simulink model "FeedForward_control"  (R2021a)
settings: Solver=VariableStepAuto  StartTime=0.0  StopTime=12.0  FixedStep=0.0001  MaxStep=0.1111111111111111  RelTol=1e-3
undefined symbols (not defined in the file): sigbuilder_block
settings Model: Creator=Mehra  LastModifiedBy=Mehra

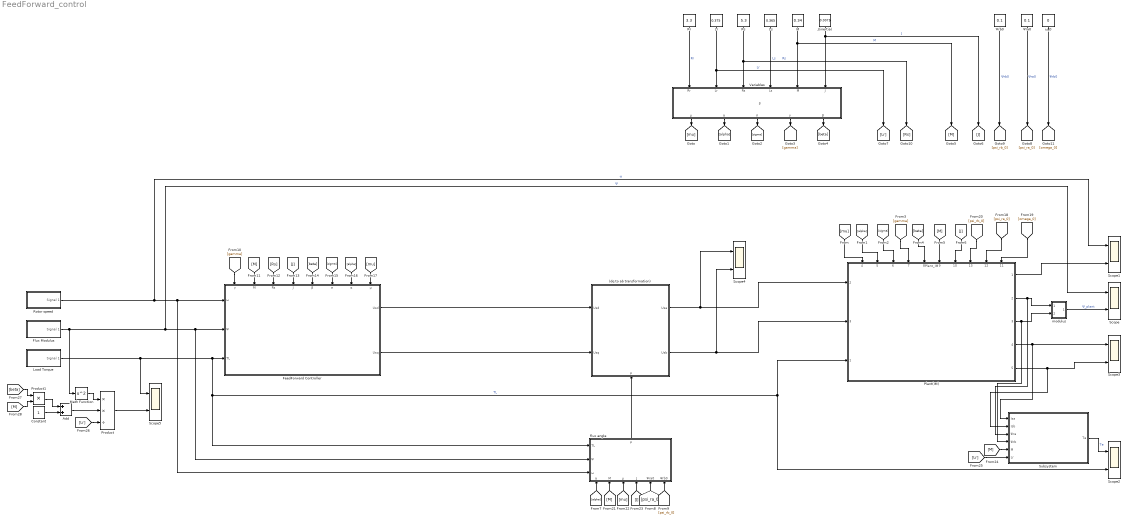
== system FeedForward_control ==
  note: β
  (dq to ab transformation) : Subsystem
      settings: PortSchema="{\"entries\":[{\"content\":{\"sides\":[{\"content\":{\"connectorIds\":[\"In1\",\"In2\"]},\"type\":\"ConnectorPlacement.EquallySpacedRectSide\",\"uuid\":\"fcc9e9c0-f3ff-45b3-b4d9-89988d9b9a34\"},{\"content\":{\"connectorIds\":[\"Out1\",\"Out2\"],\"side\":\"RIGHT\"},\"type\":\"ConnectorPlacement.EquallySpacedRectSide\",\"uuid\":\"b8117d1c-eda8-48ca-a376-b80f3451eb1b\"},{\"content\":{\"connectorIds\":[],\"side\":\"TOP\"},\"type\":\"ConnectorPlacement.EquallySpacedRectSide\",\"uuid\":\"632a2e27-4ebf-4489-a7a1-4102ed33f7de\"},{\"content\":{\"connectorIds\":[\"In3\"],\"side\":\"BOTTOM\"},\"type\":\"ConnectorPlacement.EquallySpacedRectSide\",\"uuid\":\"b1ed2b98-7899-49a7-98d1-ff7a05505f88\"}]},\"type\":\"ConnectorPlacement.EquallySpacedConnector\",\"uuid\":\"0e689d41-d128-44ad-a484-465e7f7df4f8\"}],\"packageUris\":[\"http://schema.mathworks.com/mf0/Connector/R2020b\"],\"version\":\"1.0\"}"
  Add : Sum
  Constant : Constant
  FeedForward Controller : Subsystem
      settings: PortSchema="{\"entries\":[{\"content\":{\"sides\":[{\"content\":{\"connectorIds\":[\"In1\",\"In2\",\"In3\"]},\"type\":\"ConnectorPlacement.EquallySpacedRectSide\",\"uuid\":\"d7ac22ed-73dc-4923-8a02-de2b77bc4b56\"},{\"content\":{\"connectorIds\":[\"Out1\",\"Out2\"],\"side\":\"RIGHT\"},\"type\":\"ConnectorPlacement.EquallySpacedRectSide\",\"uuid\":\"0ed82d2d-ac01-4440-b414-7b739c3193d9\"},{\"content\":{\"connectorIds\":[\"In4\",\"In5\",\"In6\",\"In7\",\"In8\",\"In9\",\"In10\",\"In11\"],\"side\":\"TOP\"},\"type\":\"ConnectorPlacement.EquallySpacedRectSide\",\"uuid\":\"be3374af-951c-49b1-9762-82694f1e2186\"}]},\"type\":\"ConnectorPlacement.EquallySpacedConnector\",\"uuid\":\"01640f11-0e41-43e3-9a6d-1e07964cb7e3\"}],\"packageUris\":[\"http://schema.mathworks.com/mf0/Connector/R2020b\"],\"version\":\"1.0\"}"
  Flux Modulus : Subsystem  Tag=STV Subsys  LoadFcn=sigbuilder_block('load');  StartFcn=sigbuilder_block('start');  StopFcn=sigbuilder_block('stop');  ClipboardFcn=sigbuilder_block('clipboard');  mask(Sigbuilder block){tuvar=[0:10]}
      mask help: Simulink:masks:SigbuilderBlock_MD
      mask init:
      | if ~strcmp(get_param(bdroot(gcbh),'SimulationStatus'),'stopped') tuvar = sigbuilder_block('maskInit'); end
      settings: CopyFcn=sigbuilder_block('copy');  DeleteFcn=sigbuilder_block('delete');  ModelCloseFcn=sigbuilder_block('modelClose');  PreSaveFcn=sigbuilder_block('preSave');  PauseFcn=sigbuilder_block('pause');  ContinueFcn=sigbuilder_block('continue');  NameChangeFcn=sigbuilder_block('namechange');  OpenFcn=sigbuilder_block('open',[433.8 177.6 550.8 400.2 ]);  CloseFcn=sigbuilder_block('close');
      mask Display: plot(0, 0, 100, 100,[2, 2, 32, 32, 2], [68, 8, 8, 68, 68],[32, 2], [38, 38], [32, 19, 2],[53, 60, 44], [32, 17, 17, 2],[16, 16, 31, 31]);txt = getActiveGroup(gcbh);text(2, 100, txt,'verticalAlignment', 'top');
  J(inertia) : Constant  Value=0.0075
  Load Torque : Subsystem  Tag=STV Subsys  LoadFcn=sigbuilder_block('load');  StartFcn=sigbuilder_block('start');  StopFcn=sigbuilder_block('stop');  ClipboardFcn=sigbuilder_block('clipboard');  mask(Sigbuilder block){tuvar=[0:10]}
      mask help: Simulink:masks:SigbuilderBlock_MD
      mask init:
      | if ~strcmp(get_param(bdroot(gcbh),'SimulationStatus'),'stopped') tuvar = sigbuilder_block('maskInit'); end
      settings: CopyFcn=sigbuilder_block('copy');  DeleteFcn=sigbuilder_block('delete');  ModelCloseFcn=sigbuilder_block('modelClose');  PreSaveFcn=sigbuilder_block('preSave');  PauseFcn=sigbuilder_block('pause');  ContinueFcn=sigbuilder_block('continue');  NameChangeFcn=sigbuilder_block('namechange');  OpenFcn=sigbuilder_block('open',[418.2 149.4 550.8 400.2 ]);  CloseFcn=sigbuilder_block('close');
      mask Display: plot(0, 0, 100, 100,[2, 2, 32, 32, 2], [68, 8, 8, 68, 68],[32, 2], [38, 38], [32, 19, 2],[53, 60, 44], [32, 17, 17, 2],[16, 16, 31, 31]);txt = getActiveGroup(gcbh);text(2, 100, txt,'verticalAlignment', 'top');
  Lr : Constant  Value=0.375
  Ls : Constant  Value=0.365
  M : Constant  Value=0.34
  Math Function : Math  Operator=square  SaturateOnIntegerOverflow=on
  Plant(IM) : ModelReference  ModelNameDialog=Plant_IM  SimulationMode=Normal  ModelReferenceVersion=1.33
      settings: PortSchema="{\"entries\":[{\"content\":{\"sides\":[{\"content\":{\"connectorIds\":[\"In2\",\"In3\",\"In1\"]},\"type\":\"ConnectorPlacement.EquallySpacedRectSide\",\"uuid\":\"c1ced4ac-9292-447b-a16b-48862d3db151\"},{\"content\":{\"connectorIds\":[\"Out1\",\"Out2\",\"Out3\",\"Out4\",\"Out5\"],\"side\":\"RIGHT\"},\"type\":\"ConnectorPlacement.EquallySpacedRectSide\",\"uuid\":\"13a72579-fb39-4c86-8f38-f8272c138e74\"},{\"content\":{\"connectorIds\":[\"In4\",\"In5\",\"In6\",\"In7\",\"In8\",\"In9\",\"In10\",\"In13\",\"In12\",\"In11\"],\"side\":\"TOP\"},\"type\":\"ConnectorPlacement.EquallySpacedRectSide\",\"uuid\":\"7112169d-3c72-435f-89ee-d1fe7807fab2\"}]},\"type\":\"ConnectorPlacement.EquallySpacedConnector\",\"uuid\":\"c43df563-9598-43b0-9064-e7550f78106e\"}],\"packageUris\":[\"http://schema.mathworks.com/mf0/Connector/R2020b\"],\"version\":\"1.0\"}"
  Product : Product  Inputs=**/
  Product1 : Product
  Rotor speed : Subsystem  Tag=STV Subsys  LoadFcn=sigbuilder_block('load');  StartFcn=sigbuilder_block('start');  StopFcn=sigbuilder_block('stop');  ClipboardFcn=sigbuilder_block('clipboard');  mask(Sigbuilder block){tuvar=[0:10]}
      mask help: Simulink:masks:SigbuilderBlock_MD
      mask init:
      | if ~strcmp(get_param(bdroot(gcbh),'SimulationStatus'),'stopped') tuvar = sigbuilder_block('maskInit'); end
      settings: CopyFcn=sigbuilder_block('copy');  DeleteFcn=sigbuilder_block('delete');  ModelCloseFcn=sigbuilder_block('modelClose');  PreSaveFcn=sigbuilder_block('preSave');  PauseFcn=sigbuilder_block('pause');  ContinueFcn=sigbuilder_block('continue');  NameChangeFcn=sigbuilder_block('namechange');  OpenFcn=sigbuilder_block('open',[418.2 149.4 550.8 400.2 ]);  CloseFcn=sigbuilder_block('close');
      mask Display: plot(0, 0, 100, 100,[2, 2, 32, 32, 2], [68, 8, 8, 68, 68],[32, 2], [38, 38], [32, 19, 2],[53, 60, 44], [32, 17, 17, 2],[16, 16, 31, 31]);txt = getActiveGroup(gcbh);text(2, 100, txt,'verticalAlignment', 'top');
  Rr : Constant  Value=3.3
  Rs : Constant  Value=5.3
  Scope{,1..5} (6 alike) : Scope  NumInputPorts=2
  Subsystem : Subsystem
  Variables : Subsystem
  flux angle : Subsystem
      settings: PortSchema="{\"entries\":[{\"content\":{\"sides\":[{\"content\":{\"connectorIds\":[\"In1\",\"In2\",\"In3\"]},\"type\":\"ConnectorPlacement.EquallySpacedRectSide\",\"uuid\":\"954ddc6c-32ec-4fca-997a-51b3ced09e6e\"},{\"content\":{\"connectorIds\":[],\"side\":\"RIGHT\"},\"type\":\"ConnectorPlacement.EquallySpacedRectSide\",\"uuid\":\"d23f0106-fd66-41c5-9167-f0bfa2e5f0d7\"},{\"content\":{\"connectorIds\":[\"Out1\"],\"side\":\"TOP\"},\"type\":\"ConnectorPlacement.EquallySpacedRectSide\",\"uuid\":\"ec2ab734-74ce-4c08-89a8-e0d0cab377a3\"},{\"content\":{\"connectorIds\":[\"In4\",\"In5\",\"In6\",\"In7\",\"In8\",\"In9\"],\"side\":\"BOTTOM\"},\"type\":\"ConnectorPlacement.EquallySpacedRectSide\",\"uuid\":\"e8fbabf1-c1e7-4b41-8038-4f25f2d2c141\"}]},\"type\":\"ConnectorPlacement.EquallySpacedConnector\",\"uuid\":\"2eb72d65-4150-4441-ba17-035a64db8a78\"}],\"packageUris\":[\"http://schema.mathworks.com/mf0/Connector/R2020b\"],\"version\":\"1.0\"}"
  modulus : Subsystem
  Ψra0 : Constant  Value=0.1
  Ψrb0 : Constant  Value=0.1
  ω_0 : Constant  Value=0
  wires:
  Rs/1 -> [Rs], Variables/3(Rs)  "Rs"
  Lr/1 -> [Lr], Variables/2(Lr)  "Lr"
  M/1 -> [M], Variables/5(M)  "M"
  Variables/1(µ) -> [mu]
  Rr/1 -> Variables/1(Rr)  "Rr"
  J(inertia)/1 -> [J], Variables/6(J)  "J"
  Ls/1 -> Variables/4(Ls)  "Ls"
  Variables/2(α) -> [alpha]
  Variables/4(γ) -> [gamma]
  [beta] -> Plant(IM)/8
  [sigma] -> Plant(IM)/6
  Variables/3(σ) -> [sigma]
  [M] -> Plant(IM)/9
  Variables/5(β) -> [beta]
  [gamma] -> Plant(IM)/7
  [alpha] -> Plant(IM)/5
  [J] -> Plant(IM)/10
  [mu] -> Plant(IM)/4
  [alpha] -> flux angle/4(α)
  [psi_ra_0] -> flux angle/8(Ψra0)
  [psi_rb_0] -> flux angle/9(Ψrb0)
  Ψrb0/1 -> [psi_rb_0]  "Ψrb0"
  Ψra0/1 -> [psi_ra_0]  "Ψra0"
  Rotor speed/1(Signal 1) -> Scope1/1, flux angle/3(ω), FeedForward Controller/1(ω)  "ω"
  Flux Modulus/1(Signal 1) -> Math Function/1, Scope/1, flux angle/2(Ψ), FeedForward Controller/2(Ψ)  "Ψ"
  Load Torque/1(Signal 1) -> Plant(IM)/1, Scope2/2, flux angle/1(TL), FeedForward Controller/3(TL), Scope5/1  "TL"
  [gamma] -> FeedForward Controller/4(γ)
  [M] -> FeedForward Controller/5(M)
  [Rs] -> FeedForward Controller/6(Rs)
  [J] -> FeedForward Controller/7(J)
  [beta] -> FeedForward Controller/8(β)
  [sigma] -> FeedForward Controller/9(σ)
  [alpha] -> FeedForward Controller/10(α)
  [mu] -> FeedForward Controller/11(µ)
  [psi_rb_0] -> Plant(IM)/13
  [psi_ra_0] -> Plant(IM)/12
  [omega_0] -> Plant(IM)/11
  ω_0/1 -> [omega_0]  "Ψrb0"
  [M] -> flux angle/5(M)
  [mu] -> flux angle/6(µ)
  [J] -> flux angle/7(J)
  FeedForward Controller/2(Usq) -> (dq to ab transformation)/2(Usq)
  flux angle/1(ρ) -> (dq to ab transformation)/3(ρ)
  (dq to ab transformation)/1(Usa) -> Scope4/1, Plant(IM)/2
  (dq to ab transformation)/2(Usb) -> Scope4/2, Plant(IM)/3
  FeedForward Controller/1(Usd) -> (dq to ab transformation)/1(Usd)
  Plant(IM)/2 -> Subsystem/3(Ψra), modulus/1(Ψra)
  Plant(IM)/3 -> Subsystem/4(Ψrb), modulus/2(Ψrb)
  modulus/1(Out1) -> Scope/2  "Ψ_plant"
  Plant(IM)/1 -> Scope1/2
  Plant(IM)/4 -> Subsystem/1(Isa), Scope3/1
  Plant(IM)/5 -> Subsystem/2(Isb), Scope3/2
  [M] -> Subsystem/5(M)
  [Lr] -> Subsystem/6(Lr)
  Subsystem/1(Te) -> Scope2/1  "Te"
  Math Function/1 -> Product/1
  [Lr] -> Product/3
  Add/1 -> Product/2
  Constant/1 -> Add/2
  Product1/1 -> Add/1
  [beta] -> Product1/1
  [M] -> Product1/2
  Product/1 -> Scope5/2

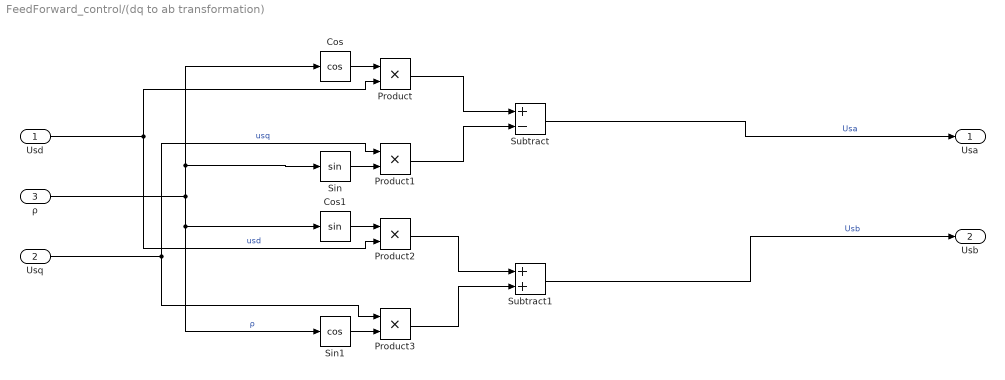
== system FeedForward_control/(dq to ab transformation) ==
  Usd : Inport
  Usq : Inport  Port=2
  ρ : Inport  Port=3
  Cos : Trigonometry  Operator=cos
  Cos1 : Trigonometry
  Product{,1..3} (4 alike) : Product
  Sin : Trigonometry
  Sin1 : Trigonometry  Operator=cos
  Subtract : Sum  Inputs=+-
  Subtract1 : Sum
  Usa : Outport
  Usb : Outport  Port=2
  wires:
  Subtract1/1 -> Usb/1  "Usb"
  Subtract/1 -> Usa/1  "Usa"
  ρ/1 -> Sin1/1, Cos1/1, Sin/1, Cos/1  "ρ"
  Cos/1 -> Product/1
  Sin/1 -> Product1/2
  Cos1/1 -> Product2/1
  Sin1/1 -> Product3/2
  Usd/1 -> Product2/2, Product/2  "usd"
  Usq/1 -> Product3/1, Product1/1  "usq"
  Product/1 -> Subtract/1
  Product1/1 -> Subtract/2
  Product2/1 -> Subtract1/1
  Product3/1 -> Subtract1/2

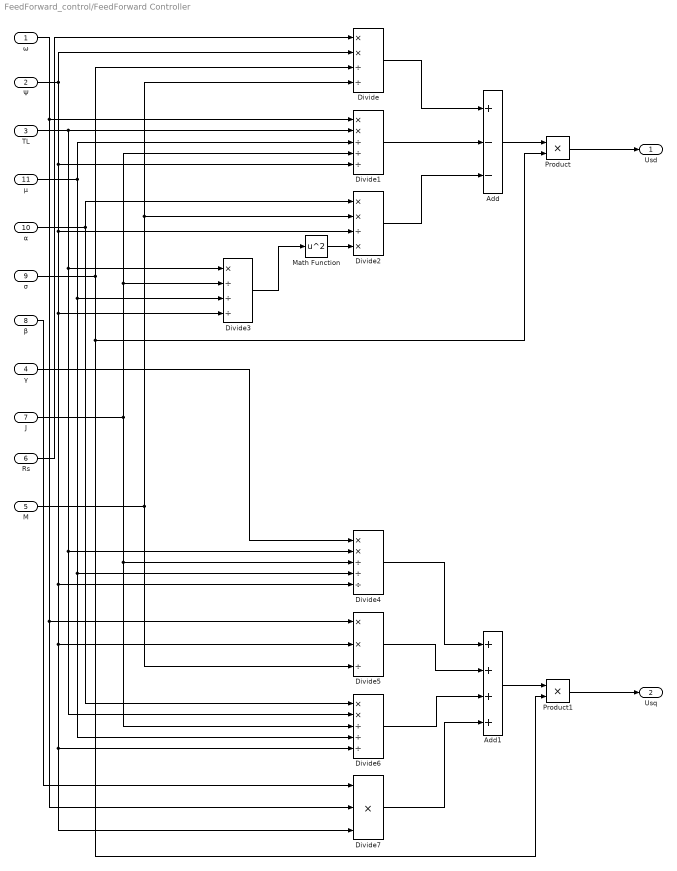
== system FeedForward_control/FeedForward Controller ==
  ω : Inport
  Ψ : Inport  Port=2
  TL : Inport  Port=3
  γ : Inport  Port=4
  M : Inport  Port=5
  Rs : Inport  Port=6
  J : Inport  Port=7
  β : Inport  Port=8
  σ : Inport  Port=9
  α : Inport  Port=10
  µ : Inport  Port=11
  Add : Sum  Inputs=+--
  Add1 : Sum  Inputs=++++
  Divide : Product  Inputs=**//
  Divide1 : Product  Inputs=**///
  Divide2 : Product  Inputs=**/*
  Divide3 : Product  Inputs=*///
  Divide4 : Product  Inputs=**///
  Divide5 : Product  Inputs=**/
  Divide6 : Product  Inputs=**///
  Divide7 : Product  Inputs=***
  Math Function : Math  Operator=square  SaturateOnIntegerOverflow=on
  Product : Product
  Product1 : Product
  Usd : Outport
  Usq : Outport  Port=2
  wires:
  α/1 -> Divide2/1, Divide6/1
  M/1 -> Divide5/3, Divide2/2, Divide/4
  J/1 -> Divide3/2, Divide1/4, Divide4/3, Divide6/3
  γ/1 -> Divide4/1
  Divide6/1 -> Add1/3
  Divide7/1 -> Add1/4
  Divide1/1 -> Add/2
  TL/1 -> Divide1/2, Divide3/1, Divide4/2, Divide6/2
  Ψ/1 -> Divide7/3, Divide6/5, Divide5/2, Divide4/5, Divide3/4, Divide2/3, Divide1/5, Divide/2
  Divide2/1 -> Add/3
  Math Function/1 -> Divide2/4
  µ/1 -> Divide1/3, Divide3/3, Divide4/4, Divide6/4
  Add1/1 -> Product1/1
  Product1/1 -> Usq/1
  Divide4/1 -> Add1/1
  Divide5/1 -> Add1/2
  ω/1 -> Divide7/2, Divide5/1, Divide1/1
  σ/1 -> Divide/3, Product1/2, Product/2
  Rs/1 -> Divide/1
  Divide3/1 -> Math Function/1
  β/1 -> Divide7/1
  Add/1 -> Product/1
  Divide/1 -> Add/1
  Product/1 -> Usd/1

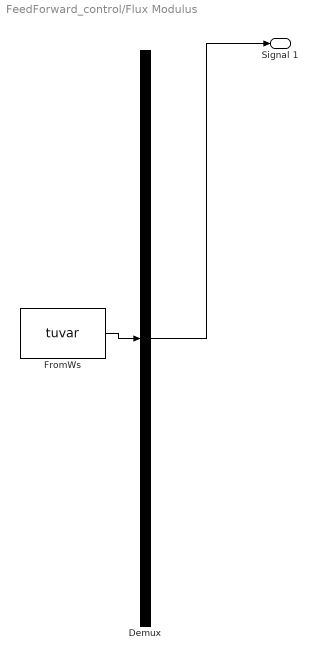
== system FeedForward_control/Flux Modulus ==
  Demux : Demux  Tag=STV Demux  Outputs=1
      settings: DisplayOption=none
  FromWs : FromWorkspace  Tag=STV FromWs  VariableName=tuvar
      SigBuilderData=|
      | common.afterFinalStr = 'Extrapolate'
      | common.sampleTime = 0
      | dataSet.timeRange = [0 10]
      | dataSet.name = 'Group 1'
      | sbobj.Groups.Name = 'Group 1'
      | sbobj.Groups.Signals.Name = 'Signal 1'
      | sbobj.Groups.Signals.XData = [0 0.32 1.5 1.8 10]
      | sbobj.Groups.Signals.YData = [0.001 1.16 1.16 0.8 0.8]
  Signal 1 : Outport  Tag=STV Outport
  wires:
  Demux/1 -> Signal 1/1
  FromWs/1 -> Demux/1

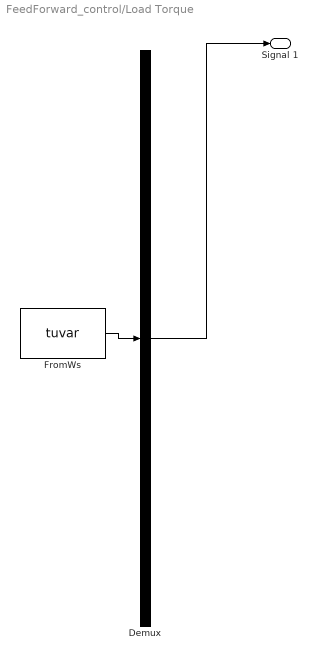
== system FeedForward_control/Load Torque ==
  Demux : Demux  Tag=STV Demux  Outputs=1
      settings: DisplayOption=none
  FromWs : FromWorkspace  Tag=STV FromWs  VariableName=tuvar
      SigBuilderData=|
      | common.afterFinalStr = 'Extrapolate'
      | common.sampleTime = 0
      | dataSet.timeRange = [0 10]
      | dataSet.name = 'Group 1'
      | sbobj.Groups.Name = 'Group 1'
      | sbobj.Groups.Signals.Name = 'Signal 1'
      | sbobj.Groups.Signals.XData = [0 0.32 0.32 1 1 10]
      | sbobj.Groups.Signals.YData = [0 0 5.8 5.8 4.8 4.8]
  Signal 1 : Outport  Tag=STV Outport
  wires:
  Demux/1 -> Signal 1/1
  FromWs/1 -> Demux/1

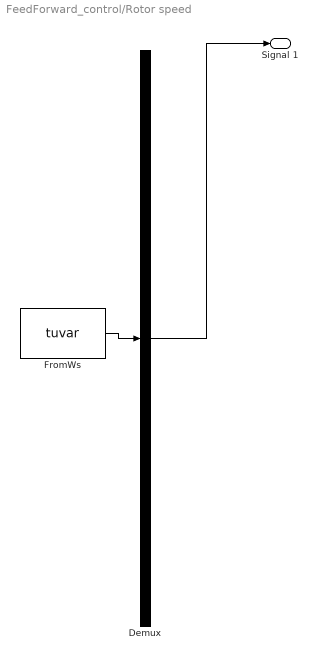
== system FeedForward_control/Rotor speed ==
  Demux : Demux  Tag=STV Demux  Outputs=1
      settings: DisplayOption=none
  FromWs : FromWorkspace  Tag=STV FromWs  VariableName=tuvar
      SigBuilderData=|
      | common.afterFinalStr = 'Extrapolate'
      | common.sampleTime = 0
      | dataSet.timeRange = [0 10]
      | dataSet.name = 'Group 1'
      | sbobj.Groups.Name = 'Group 1'
      | sbobj.Groups.Signals.Name = 'Signal 1'
      | sbobj.Groups.Signals.XData = [0 0.32 1 10]
      | sbobj.Groups.Signals.YData = [0 0 -100 -100]
  Signal 1 : Outport  Tag=STV Outport
  wires:
  Demux/1 -> Signal 1/1
  FromWs/1 -> Demux/1

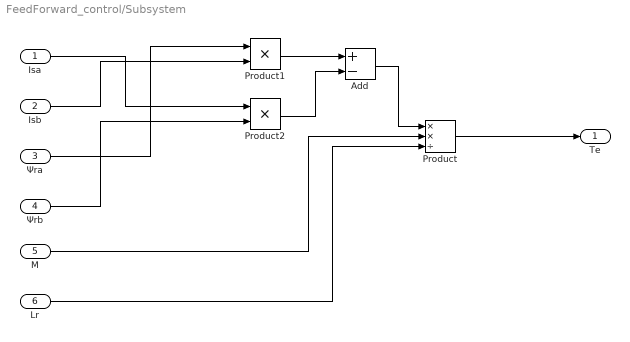
== system FeedForward_control/Subsystem ==
  Isa : Inport
  Isb : Inport  Port=2
  Ψra : Inport  Port=3
  Ψrb : Inport  Port=4
  M : Inport  Port=5
  Lr : Inport  Port=6
  Add : Sum  Inputs=+-
  Product : Product  Inputs=**/
  Product1 : Product
  Product2 : Product
  Te : Outport
  wires:
  Product/1 -> Te/1
  Add/1 -> Product/1
  M/1 -> Product/2
  Lr/1 -> Product/3
  Product1/1 -> Add/1
  Product2/1 -> Add/2
  Ψra/1 -> Product1/1
  Isb/1 -> Product1/2
  Ψrb/1 -> Product2/2
  Isa/1 -> Product2/1

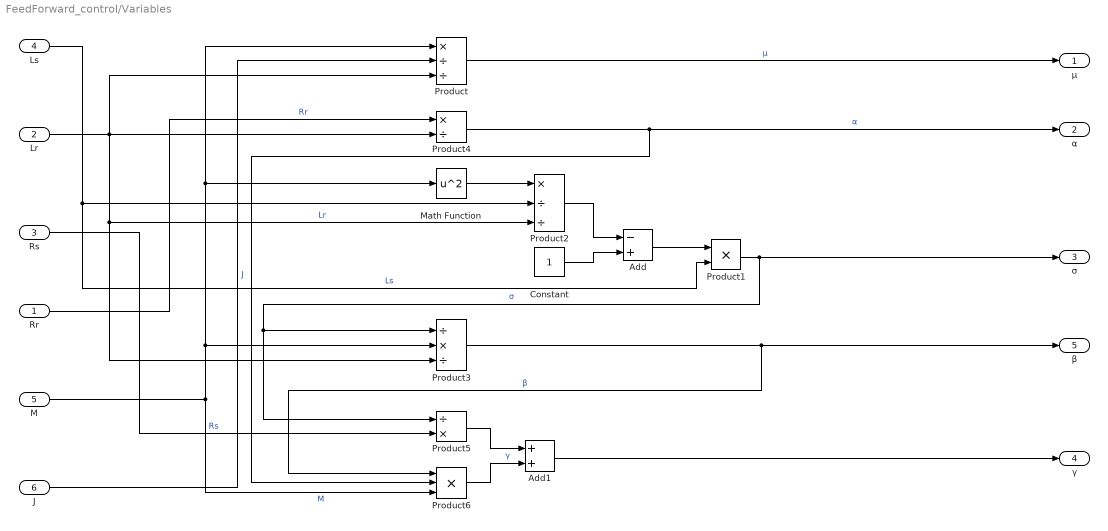
== system FeedForward_control/Variables ==
  Rr : Inport
  Lr : Inport  Port=2
  Rs : Inport  Port=3
  Ls : Inport  Port=4
  M : Inport  Port=5
  J : Inport  Port=6
  Add : Sum  Inputs=-+
  Add1 : Sum
  Constant : Constant
  Math Function : Math  Operator=square  SaturateOnIntegerOverflow=on
  Product : Product  Inputs=*//
  Product1 : Product
  Product2 : Product  Inputs=*//
  Product3 : Product  Inputs=/*/
  Product4 : Product  Inputs=*/
  Product5 : Product  Inputs=/*
  Product6 : Product  Inputs=3
  µ : Outport
  α : Outport  Port=2
  σ : Outport  Port=3
  γ : Outport  Port=4
  β : Outport  Port=5
  wires:
  M/1 -> Product3/2, Math Function/1, Product/1, Product6/3  "M"
  J/1 -> Product/2  "J"
  Lr/1 -> Product4/2, Product/3, Product2/3, Product3/3  "Lr"
  Product/1 -> µ/1  "µ"
  Add/1 -> Product1/1
  Ls/1 -> Product2/2, Product1/2  "Ls"
  Product1/1 -> Product3/1, Product5/1, σ/1  "σ"
  Constant/1 -> Add/2
  Product2/1 -> Add/1
  Math Function/1 -> Product2/1
  Product3/1 -> Product6/1, β/1  "β"
  Rr/1 -> Product4/1  "Rr"
  Product4/1 -> Product6/2, α/1  "α"
  Rs/1 -> Product5/2  "Rs"
  Product6/1 -> Add1/2  "γ"
  Product5/1 -> Add1/1
  Add1/1 -> γ/1

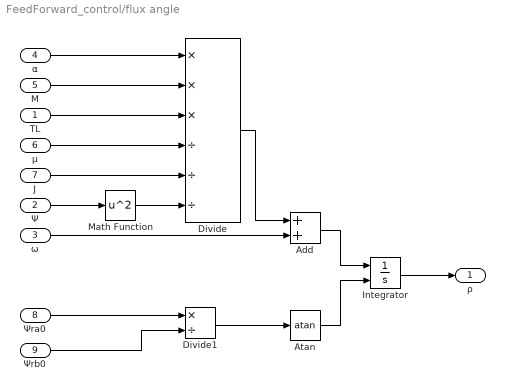
== system FeedForward_control/flux angle ==
  TL : Inport
  Ψ : Inport  Port=2
  ω : Inport  Port=3
  α : Inport  Port=4
  M : Inport  Port=5
  µ : Inport  Port=6
  J : Inport  Port=7
  Ψra0 : Inport  Port=8
  Ψrb0 : Inport  Port=9
  Add : Sum
  Atan : Trigonometry  Operator=atan
  Divide : Product  Inputs=***///
  Divide1 : Product  Inputs=*/
  Integrator : Integrator  InitialConditionSource=external
  Math Function : Math  Operator=square  SaturateOnIntegerOverflow=on
  ρ : Outport
  wires:
  Add/1 -> Integrator/1
  Integrator/1 -> ρ/1
  ω/1 -> Add/2
  Ψ/1 -> Math Function/1
  α/1 -> Divide/1
  Ψrb0/1 -> Divide1/2
  Ψra0/1 -> Divide1/1
  Divide1/1 -> Atan/1
  Divide/1 -> Add/1
  Atan/1 -> Integrator/2
  Math Function/1 -> Divide/6
  TL/1 -> Divide/3
  M/1 -> Divide/2
  µ/1 -> Divide/4
  J/1 -> Divide/5

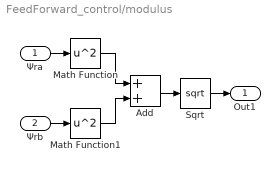
== system FeedForward_control/modulus ==
  Ψra : Inport
  Ψrb : Inport  Port=2
  Add : Sum
  Math Function : Math  Operator=square  SaturateOnIntegerOverflow=on
  Math Function1 : Math  Operator=square  SaturateOnIntegerOverflow=on
  Sqrt : Sqrt  SaturateOnIntegerOverflow=on
  Out1 : Outport
  wires:
  Ψrb/1 -> Math Function1/1
  Math Function1/1 -> Add/2
  Add/1 -> Sqrt/1
  Ψra/1 -> Math Function/1
  Math Function/1 -> Add/1
  Sqrt/1 -> Out1/1
